simulink model "WIper_Project"  (R2021a)
settings: Solver=FixedStepDiscrete  StartTime=0.0  StopTime=20  FixedStep=0.01  RelTol=1e-3
undefined symbols (not defined in the file): sigbuilder_block
libraries: simulink x1
settings Model: Creator=Beshary  LastModifiedBy=Beshary
settings OptimizationCC: DefaultParameterBehavior=Inlined  UseDivisionForNetSlopeComputation=on  GainParamInheritBuiltInType=on  UseFloatMulNetSlope=on  InlineInvariantSignals=on  PassReuseOutputArgsAs=Individual arguments  ZeroExternalMemoryAtStartup=off  ZeroInternalMemoryAtStartup=off  NoFixptDivByZeroProtection=on  EfficientFloat2IntCast=on  LifeSpan=1  OptimizeBlockOrder=speed  DifferentSizesBufferReuse=on  EfficientTunableParamExpr=on
settings DebuggingCC: ParameterTunabilityLossMsg=error
settings HardwareCC: ProdLongLongMode=on
settings SFSimCC: MATLABDynamicMemAlloc=off
settings RTWCC: SystemTargetFile=ert.tlc  TemplateMakefile=ert_default_tmf
settings CodeAppCC: ForceParamTrailComments=on  IgnoreCustomStorageClasses=off  OperatorAnnotations=on  SimulinkDataObjDesc=on  SFDataObjDesc=on  CustomSymbolStrGlobalVar=rt$N$M  CustomSymbolStrType=$N$M  CustomSymbolStrFcn=$N$M$F  CustomSymbolStrMacro=$N$M  InsertBlockDesc=on
settings ERTTargetCC: TargetLangStandard=C99 (ISO)  GenerateSampleERTMain=on  IncludeMdlTerminateFcn=off  CombineSignalStateStructs=on  SupportComplex=off  SupportNonInlinedSFcns=on  InlinedParameterPlacement=NonHierarchical  ERTCustomFileTemplate=example_file_process.tlc  ERTFilePackagingFormat=CompactWithDataFile

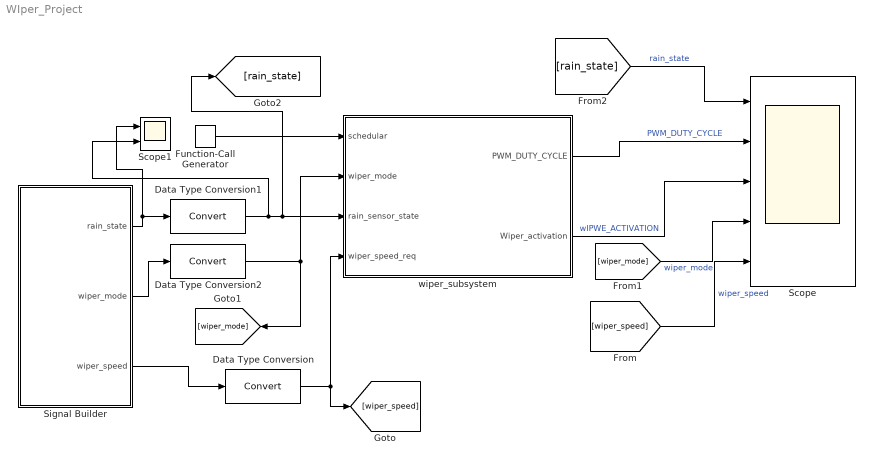
== system WIper_Project ==
  Data Type Conversion : DataTypeConversion
  Data Type Conversion1 : DataTypeConversion
  Data Type Conversion2 : DataTypeConversion
  Function-Call Generator : simulink/Ports & Subsystems/Function-Call Generator  sample_time=0.01  numberOfIterations=1  DisallowWideOutput=off
  Scope : Scope  NumInputPorts=5
  Scope1 : Scope  NumInputPorts=2
  Signal Builder : Subsystem  Tag=STV Subsys  LoadFcn=sigbuilder_block('load',[5.4 30 1141.2 522.6 ]);  StartFcn=sigbuilder_block('start');  StopFcn=sigbuilder_block('stop');  ClipboardFcn=sigbuilder_block('clipboard');  mask(Sigbuilder block){tuvar=[0:10]}
      mask help: Simulink:masks:SigbuilderBlock_MD
      mask init:
      | if ~strcmp(get_param(bdroot(gcbh),'SimulationStatus'),'stopped') tuvar = sigbuilder_block('maskInit'); end
      settings: CopyFcn=sigbuilder_block('copy');  DeleteFcn=sigbuilder_block('delete');  ModelCloseFcn=sigbuilder_block('modelClose');  PreSaveFcn=sigbuilder_block('preSave');  PauseFcn=sigbuilder_block('pause');  ContinueFcn=sigbuilder_block('continue');  NameChangeFcn=sigbuilder_block('namechange');  OpenFcn=sigbuilder_block('open',[5.4 30 1141.2 522.6 ]);  CloseFcn=sigbuilder_block('close');
      mask Display: plot(0, 0, 100, 100,[2, 2, 32, 32, 2], [68, 8, 8, 68, 68],[32, 2], [38, 38], [32, 19, 2],[53, 60, 44], [32, 17, 17, 2],[16, 16, 31, 31]);txt = getActiveGroup(gcbh);text(2, 100, txt,'verticalAlignment', 'top');
  wiper_subsystem : Subsystem
  wires:
  Function-Call Generator/1 -> wiper_subsystem/1(schedular)
  wiper_subsystem/1(PWM_DUTY_CYCLE) -> Scope/2  "PWM_DUTY_CYCLE"
  wiper_subsystem/2(Wiper_activation) -> Scope/3  "wIPWE_ACTIVATION"
  Signal Builder/2(wiper_mode) -> Data Type Conversion2/1
  Data Type Conversion2/1 -> [wiper_mode], wiper_subsystem/2(wiper_mode)
  Signal Builder/1(rain_state) -> Scope1/1, Data Type Conversion1/1
  Data Type Conversion1/1 -> Scope1/2, [rain_state], wiper_subsystem/3(rain_sensor_state)
  Signal Builder/3(wiper_speed) -> Data Type Conversion/1
  Data Type Conversion/1 -> wiper_subsystem/4(wiper_speed_req), [wiper_speed]
  [wiper_speed] -> Scope/5  "wiper_speed"
  [wiper_mode] -> Scope/4  "wiper_mode"
  [rain_state] -> Scope/1  "rain_state"

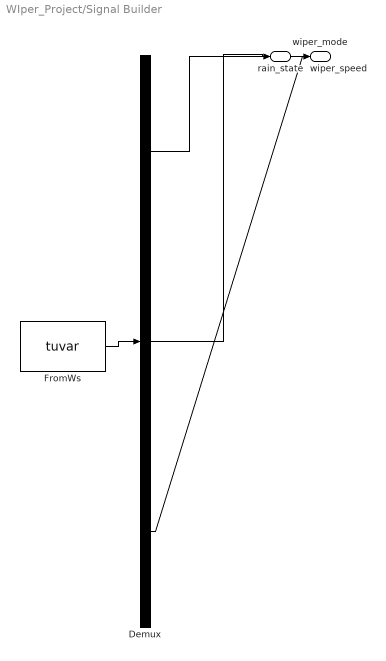
== system WIper_Project/Signal Builder ==
  Demux : Demux  Tag=STV Demux  Outputs=3
      settings: DisplayOption=none
  FromWs : FromWorkspace  Tag=STV FromWs  VariableName=tuvar
      SigBuilderData=|
      | common.afterFinalStr = 'Extrapolate'
      | common.sampleTime = 0
      | dataSet.timeRange = [0 20]
      | dataSet.name = 'Group 1'
      | sbobj.Groups.Name = 'Group 1'
      | sbobj.Groups.Signals(1).Name = 'rain_state'
      | sbobj.Groups.Signals(1).XData = [0 4 6 14 15 16 20]
      | sbobj.Groups.Signals(1).YData = [0 0 0 0 1 0 0]
      | sbobj.Groups.Signals(2).Name = 'wiper_mode'
      | sbobj.Groups.Signals(2).XData = [0 1 2 3 4 5 6 7 8 9 10 11 12 13 14 15 16 17 18 19 20]
      | sbobj.Groups.Signals(2).YData = [0 0 2 2 3 3 1 1 1 1 1 1 1 1 1 1 1 1 1 1 1]
      | sbobj.Groups.Signals(3).Name = 'wiper_speed'
      | sbobj.Groups.Signals(3).XData = [0 7 13.98 20]
      | sbobj.Groups.Signals(3).YData = [0 0 7 7]
      | sbobj.Groups.TimeRange = [0 20]
  rain_state : Outport  Tag=STV Outport
  wiper_mode : Outport  Tag=STV Outport  Port=2
  wiper_speed : Outport  Tag=STV Outport  Port=3
  wires:
  Demux/1 -> rain_state/1
  FromWs/1 -> Demux/1
  Demux/2 -> wiper_mode/1
  Demux/3 -> wiper_speed/1

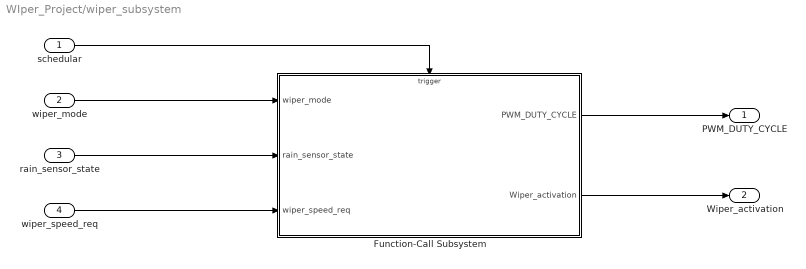
== system WIper_Project/wiper_subsystem ==
  schedular : Inport
  wiper_mode : Inport  Port=2  OutDataTypeStr=uint8
  rain_sensor_state : Inport  Port=3  OutDataTypeStr=boolean
  wiper_speed_req : Inport  Port=4  OutDataTypeStr=uint8
  Function-Call Subsystem : Subsystem  TreatAsAtomicUnit=on
  PWM_DUTY_CYCLE : Outport  OutDataTypeStr=single
  Wiper_activation : Outport  Port=2  OutDataTypeStr=boolean
  wires:
  schedular/1 -> Function-Call Subsystem/Trigger
  wiper_mode/1 -> Function-Call Subsystem/1(wiper_mode)
  rain_sensor_state/1 -> Function-Call Subsystem/2(rain_sensor_state)
  wiper_speed_req/1 -> Function-Call Subsystem/3(wiper_speed_req)
  Function-Call Subsystem/1(PWM_DUTY_CYCLE) -> PWM_DUTY_CYCLE/1
  Function-Call Subsystem/2(Wiper_activation) -> Wiper_activation/1

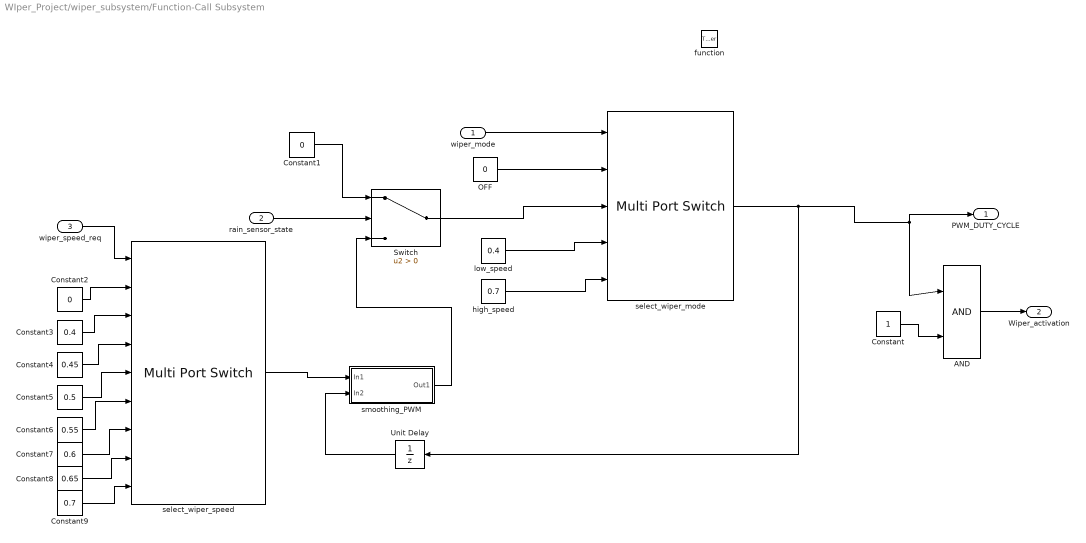
== system WIper_Project/wiper_subsystem/Function-Call Subsystem ==
  wiper_mode : Inport
  rain_sensor_state : Inport  Port=2  OutDataTypeStr=boolean
  wiper_speed_req : Inport  Port=3
  function : TriggerPort  TriggerType=function-call  VariantControl=(inherit)
  AND : Logic  IconShape=distinctive  AllPortsSameDT=off  OutDataTypeStr=boolean
  Constant : Constant
  Constant1 : Constant  Value=0
  Constant2 : Constant  Value=0
  Constant3 : Constant  Value=0.4
  Constant4 : Constant  Value=0.45
  Constant5 : Constant  Value=0.5
  Constant6 : Constant  Value=0.55
  Constant7 : Constant  Value=0.6
  Constant8 : Constant  Value=0.65
  Constant9 : Constant  Value=0.7
  OFF : Constant  Value=0
  Switch : Switch  Criteria=u2 > Threshold
  Unit Delay : UnitDelay  SampleTime=-1  HasFrameUpgradeWarning=on
  high_speed : Constant  Value=0.7
  low_speed : Constant  Value=0.4
  select_wiper_mode : MultiPortSwitch  DataPortOrder=Zero-based contiguous  Inputs=4  zeroidx=on  OutDataTypeStr=single
  select_wiper_speed : MultiPortSwitch  DataPortOrder=Zero-based contiguous  Inputs=8  zeroidx=on  OutDataTypeStr=single
  smoothing_PWM : Subsystem
  PWM_DUTY_CYCLE : Outport
  Wiper_activation : Outport  Port=2
  wires:
  wiper_mode/1 -> select_wiper_mode/1
  OFF/1 -> select_wiper_mode/2
  low_speed/1 -> select_wiper_mode/4
  high_speed/1 -> select_wiper_mode/5
  select_wiper_mode/1 -> Unit Delay/1, PWM_DUTY_CYCLE/1, AND/1
  AND/1 -> Wiper_activation/1
  Constant/1 -> AND/2
  rain_sensor_state/1 -> Switch/2
  Constant1/1 -> Switch/1
  wiper_speed_req/1 -> select_wiper_speed/1
  Constant2/1 -> select_wiper_speed/2
  Constant3/1 -> select_wiper_speed/3
  Constant9/1 -> select_wiper_speed/9
  Constant8/1 -> select_wiper_speed/8
  Constant7/1 -> select_wiper_speed/7
  Constant6/1 -> select_wiper_speed/6
  Constant5/1 -> select_wiper_speed/5
  Constant4/1 -> select_wiper_speed/4
  select_wiper_speed/1 -> smoothing_PWM/1(In1)
  Unit Delay/1 -> smoothing_PWM/2(In2)
  smoothing_PWM/1(Out1) -> Switch/3
  Switch/1 -> select_wiper_mode/3

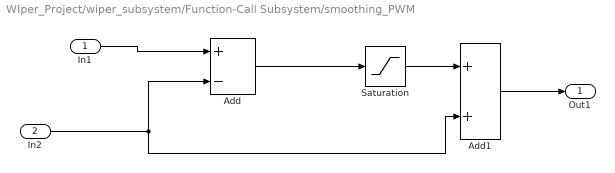
== system WIper_Project/wiper_subsystem/Function-Call Subsystem/smoothing_PWM ==
  In1 : Inport
  In2 : Inport  Port=2
  Add : Sum  Inputs=+-
  Add1 : Sum
  Saturation : Saturate  UpperLimit=0.005  LowerLimit=-0.005
  Out1 : Outport
  wires:
  In1/1 -> Add/1
  In2/1 -> Add1/2, Add/2
  Add/1 -> Saturation/1
  Saturation/1 -> Add1/1
  Add1/1 -> Out1/1
